simulink model "oneDsingleRotor"  (R2020a)
settings: Solver=VariableStepAuto  StartTime=0.0  StopTime=10.0  RelTol=1e-3
settings Model: Creator=Cyand  LastModifiedBy=Cyand

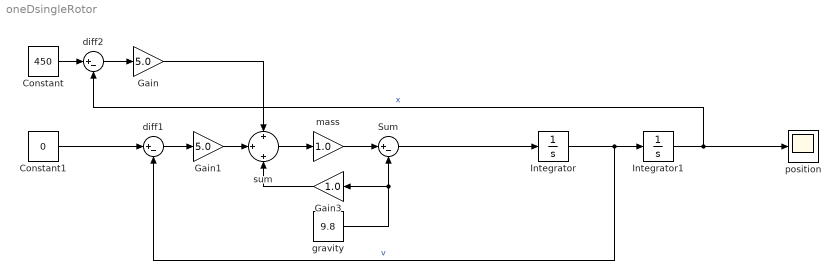
== system oneDsingleRotor ==
  Constant : Constant  Value=450
  Constant1 : Constant  Value=0
  Gain : Gain  Gain=5.0
  Gain1 : Gain  Gain=5.0
  Gain3 : Gain  Gain=1.0
  Integrator : Integrator
  Integrator1 : Integrator  InitialCondition=500
  Sum : Sum  Inputs=|+-
  diff1 : Sum  Inputs=|+-
  diff2 : Sum  Inputs=|+-
  gravity : Constant  Value=9.8
  mass : Gain  Gain=1.0
  position : Scope
  sum : Sum  Inputs=+|+|+
  wires:
  Integrator/1 -> diff1/2, Integrator1/1  "v"
  Constant1/1 -> diff1/1
  Constant/1 -> diff2/1
  Integrator1/1 -> position/1, diff2/2  "x"
  diff2/1 -> Gain/1
  diff1/1 -> Gain1/1
  Gain1/1 -> sum/2
  Gain/1 -> sum/1
  sum/1 -> mass/1
  gravity/1 -> Sum/2, Gain3/1
  mass/1 -> Sum/1
  Sum/1 -> Integrator/1
  Gain3/1 -> sum/3
